simulink subsystem "SubSystemVereinzelung"  (R2020b)
settings: Solver=VariableStepAuto  StartTime=0.0  StopTime=10.0  RelTol=1e-3
libraries: simulink x6, eeGeneralControl x5
settings Model: Creator=kaebi  LastModifiedBy=kaebi

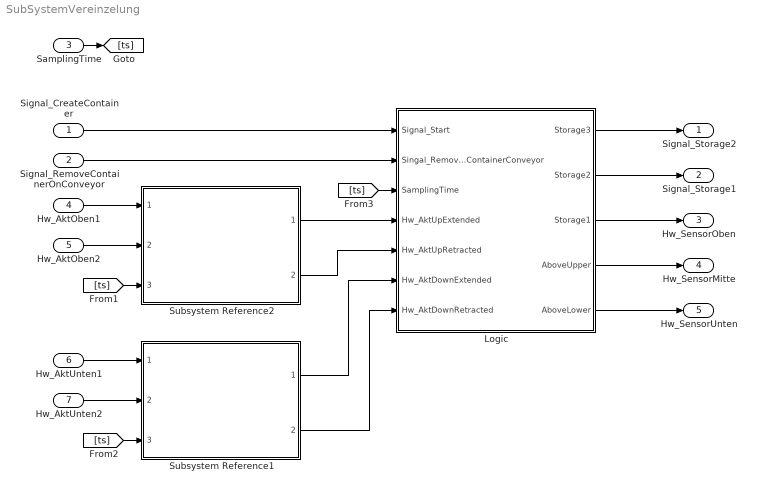
== system SubSystemVereinzelung ==
  Signal_CreateContainer : Inport
  Signal_RemoveContainerOnConveyor : Inport  Port=2
  SamplingTime : Inport  Port=3
  Hw_AktOben1 : Inport  Port=4
  Hw_AktOben2 : Inport  Port=5
  Hw_AktUnten1 : Inport  Port=6
  Hw_AktUnten2 : Inport  Port=7
  Logic : Subsystem
  Subsystem Reference1 : Subsystem  ReferencedSubsystem=SubSystemHubmagnetVereinzelung
  Subsystem Reference2 : Subsystem  ReferencedSubsystem=SubSystemHubmagnetVereinzelung
  Signal_Storage2 : Outport
  Signal_Storage1 : Outport  Port=2
  Hw_SensorOben : Outport  Port=3
  Hw_SensorMitte : Outport  Port=4
  Hw_SensorUnten : Outport  Port=5
  wires:
  Hw_AktOben1/1 -> Subsystem Reference2/1
  Hw_AktUnten1/1 -> Subsystem Reference1/1
  [ts] -> Subsystem Reference2/3
  [ts] -> Subsystem Reference1/3
  SamplingTime/1 -> [ts]
  Logic/5(AboveLower) -> Hw_SensorUnten/1
  Logic/4(AboveUpper) -> Hw_SensorMitte/1
  Logic/3(Storage1) -> Hw_SensorOben/1
  Logic/2(Storage2) -> Signal_Storage1/1
  Logic/1(Storage3) -> Signal_Storage2/1
  Signal_CreateContainer/1 -> Logic/1(Signal_Start)
  [ts] -> Logic/3(SamplingTime)
  Signal_RemoveContainerOnConveyor/1 -> Logic/2(Singal_RemoveContainerConveyor)
  Hw_AktUnten2/1 -> Subsystem Reference1/2
  Hw_AktOben2/1 -> Subsystem Reference2/2
  Subsystem Reference2/1 -> Logic/4(Hw_AktUpExtended)
  Subsystem Reference2/2 -> Logic/5(Hw_AktUpRetracted)
  Subsystem Reference1/1 -> Logic/6(Hw_AktDownExtended)
  Subsystem Reference1/2 -> Logic/7(Hw_AktDownRetracted)

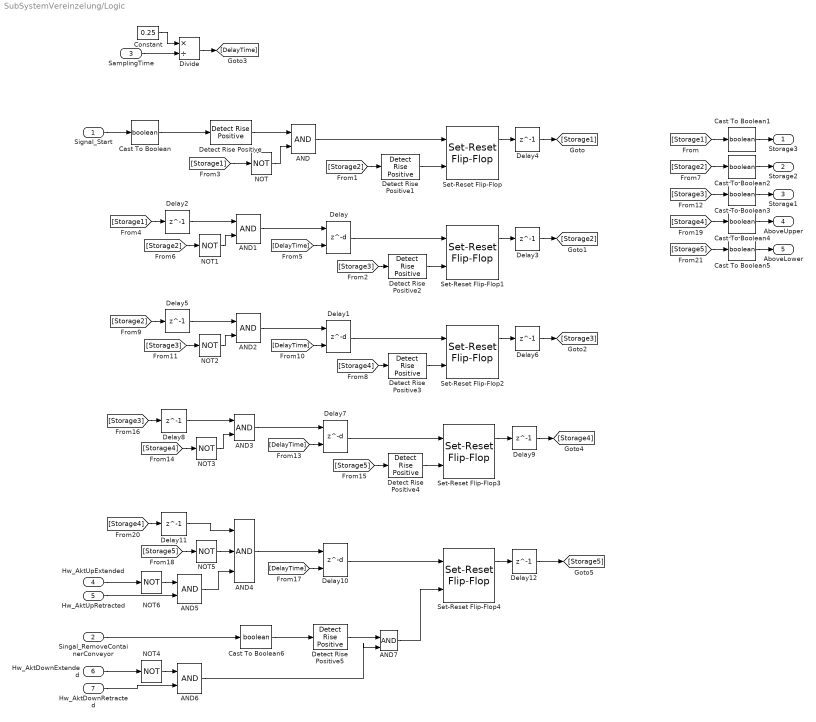
== system SubSystemVereinzelung/Logic ==
  Signal_Start : Inport
  Singal_RemoveContainerConveyor : Inport  Port=2
  SamplingTime : Inport  Port=3
  Hw_AktUpExtended : Inport  Port=4
  Hw_AktUpRetracted : Inport  Port=5
  Hw_AktDownExtended : Inport  Port=6
  Hw_AktDownRetracted : Inport  Port=7
  AND{,1..3,5..7} (7 alike) : Logic  IconShape=distinctive  AllPortsSameDT=off  OutDataTypeStr=boolean
  AND4 : Logic  Inputs=3  IconShape=distinctive  AllPortsSameDT=off  OutDataTypeStr=boolean
  Cast To Boolean{,1..6} (7 alike) : DataTypeConversion  OutDataTypeStr=boolean
  Constant : Constant  Value=0.25
  Delay{,1,7,10} (4 alike) : Delay  DelayLengthSource=Input port  DelayLengthUpperLimit=2500
      settings: InputPortMap=u0,p1
  Delay{2..6,8..9,11..12} (9 alike) : Delay  DelayLength=1
  Detect Rise Positive{,1..5} (6 alike) : simulink/Logic and Bit Operations/Detect Rise Positive  vinit=0  OutDataTypeStr=boolean
  Divide : Product  Inputs=*/
  NOT{,1..6} (7 alike) : Logic  Operator=NOT  IconShape=distinctive  AllPortsSameDT=off  OutDataTypeStr=boolean
  Set-Reset Flip-Flop{,1..4} (5 alike) : eeGeneralControl/Set-Reset Flip-Flop  LabelModeActiveChoice=Discrete  UndefState=Set  Q0=0  Ts=-1
      settings: SourceProductBaseCode=PS
  Storage3 : Outport
  Storage2 : Outport  Port=2
  Storage1 : Outport  Port=3
  AboveUpper : Outport  Port=4
  AboveLower : Outport  Port=5
  wires:
  AND6/1 -> AND7/2
  Hw_AktDownRetracted/1 -> AND6/2
  NOT4/1 -> AND6/1
  Hw_AktUpRetracted/1 -> AND5/2
  NOT6/1 -> AND5/1
  AND5/1 -> AND4/3
  Detect Rise Positive5/1 -> AND7/1
  AND7/1 -> Set-Reset Flip-Flop4/2
  Hw_AktDownExtended/1 -> NOT4/1
  Cast To Boolean/1 -> Detect Rise Positive/1
  [Storage4] -> Detect Rise Positive3/1
  Detect Rise Positive3/1 -> Set-Reset Flip-Flop2/2
  Detect Rise Positive2/1 -> Set-Reset Flip-Flop1/2
  [Storage3] -> Detect Rise Positive2/1
  Detect Rise Positive1/1 -> Set-Reset Flip-Flop/2
  [Storage2] -> Detect Rise Positive1/1
  Detect Rise Positive4/1 -> Set-Reset Flip-Flop3/2
  [Storage5] -> Detect Rise Positive4/1
  [Storage4] -> Delay11/1
  [DelayTime] -> Delay10/2
  Delay11/1 -> AND4/1
  AND4/1 -> Delay10/1
  NOT5/1 -> AND4/2
  [Storage5] -> NOT5/1
  Delay10/1 -> Set-Reset Flip-Flop4/1
  Delay12/1 -> [Storage5]
  Set-Reset Flip-Flop4/1 -> Delay12/1
  Hw_AktUpExtended/1 -> NOT6/1
  Set-Reset Flip-Flop3/1 -> Delay9/1
  Delay9/1 -> [Storage4]
  Delay7/1 -> Set-Reset Flip-Flop3/1
  [Storage4] -> NOT3/1
  NOT3/1 -> AND3/2
  AND3/1 -> Delay7/1
  Delay8/1 -> AND3/1
  [DelayTime] -> Delay7/2
  [Storage3] -> Delay8/1
  [Storage2] -> Delay5/1
  [DelayTime] -> Delay1/2
  Delay5/1 -> AND2/1
  AND2/1 -> Delay1/1
  NOT2/1 -> AND2/2
  [Storage3] -> NOT2/1
  Delay1/1 -> Set-Reset Flip-Flop2/1
  Delay6/1 -> [Storage3]
  Set-Reset Flip-Flop2/1 -> Delay6/1
  Set-Reset Flip-Flop1/1 -> Delay3/1
  Delay3/1 -> [Storage2]
  Delay4/1 -> [Storage1]
  Delay/1 -> Set-Reset Flip-Flop1/1
  [Storage2] -> NOT1/1
  NOT1/1 -> AND1/2
  AND1/1 -> Delay/1
  Delay2/1 -> AND1/1
  [DelayTime] -> Delay/2
  [Storage1] -> Delay2/1
  Divide/1 -> [DelayTime]
  [Storage1] -> NOT/1
  AND/1 -> Set-Reset Flip-Flop/1
  Set-Reset Flip-Flop/1 -> Delay4/1
  SamplingTime/1 -> Divide/2
  Constant/1 -> Divide/1
  NOT/1 -> AND/2
  Detect Rise Positive/1 -> AND/1
  Signal_Start/1 -> Cast To Boolean/1
  [Storage1] -> Cast To Boolean1/1
  Cast To Boolean1/1 -> Storage3/1
  [Storage5] -> Cast To Boolean5/1
  [Storage4] -> Cast To Boolean4/1
  [Storage3] -> Cast To Boolean3/1
  [Storage2] -> Cast To Boolean2/1
  Cast To Boolean2/1 -> Storage2/1
  Cast To Boolean3/1 -> Storage1/1
  Cast To Boolean4/1 -> AboveUpper/1
  Cast To Boolean5/1 -> AboveLower/1
  Cast To Boolean6/1 -> Detect Rise Positive5/1
  Singal_RemoveContainerConveyor/1 -> Cast To Boolean6/1
